simulink model "Trap_Model"  (R2019a)
settings: Solver=FixedStepAuto  StartTime=0.0  StopTime=3  FixedStep=dt  RelTol=1e-3
values from neighbouring files (symbols this model uses):
  disable_droplet_faults = 1    [initTrapModel.m]
  phase_1 = 0    [initMonteCarlo.m]    (also in initTrapModel.m)
  phase_2 = 0.005    [initMonteCarlo.m]    (also in initTrapModel.m)
  Q1 = 0.5*60*1000000000    (= 30000000000)    [initMonteCarlo.m]    (also in initRealModel.m = 2000; initTrapModel.m)
  Q2 = 0.5*60*1000000000    (= 30000000000)    [initMonteCarlo.m]    (also in initRealModel.m = 2000; initTrapModel.m)
  rate_1 = 0.01    [initMonteCarlo.m]    (also in initTrapModel.m)
  rate_2 = 0.01    [initMonteCarlo.m]    (also in initTrapModel.m)
  seed_1 = 0    [initMonteCarlo.m]    (also in initRealModel.m; initTrapModel.m)
  seed_2 = 1    [initMonteCarlo.m]    (also in initRealModel.m; initTrapModel.m)
libraries: simulink x4, SinglePipe_lib x3, Trap_lib x2, Junction_Lib x1
settings Model: Creator=Forest Song  LastModifiedBy=martin

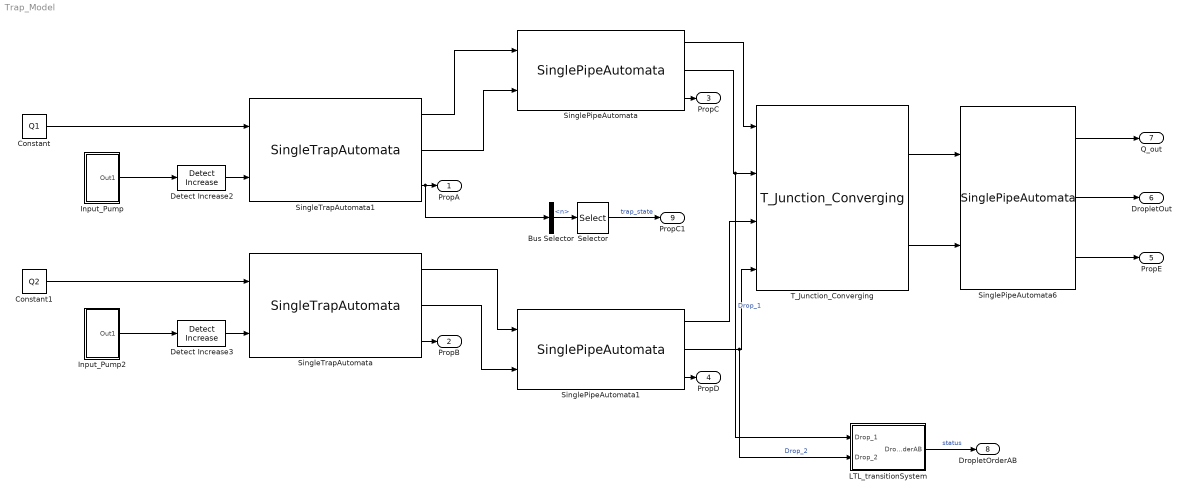
== system Trap_Model ==
  Bus Selector : BusSelector  OutputSignals=n
  Constant : Constant  Value=Q1
  Constant1 : Constant  Value=Q2
  Detect Increase2 : simulink/Logic and Bit Operations/Detect Increase  vinit=0  OutDataTypeStr=boolean
  Detect Increase3 : simulink/Logic and Bit Operations/Detect Increase  vinit=0  OutDataTypeStr=boolean
  Input_Pump : Subsystem  mask{Period=rate_1, Seed=seed_1, PhaseDelay=phase_1}
      mask prompts: Period "droplet rate"; Seed "Simulink:blkprm_prompts:RandNumInitSeed"; PhaseDelay "Simulink:blkprm_prompts:PulseContPhaseDelay"
      mask TypeOptions Period:
      | Pulse
      | Generator/Period
      mask TypeOptions Seed:
      | Uniform Random
      | Number4/Seed
      mask TypeOptions PhaseDelay:
      | Pulse
      | Generator/PhaseDelay
      mask DialogControl Seed Prompt: Seed:
      mask DialogControl PhaseDelay Prompt: Phase delay (secs):
  Input_Pump2 : Subsystem  mask{Period=rate_2, Seed=seed_2, PhaseDelay=phase_2}
      mask prompts: Period "droplet rate"; Seed "Simulink:blkprm_prompts:RandNumInitSeed"; PhaseDelay "Simulink:blkprm_prompts:PulseContPhaseDelay"
      mask TypeOptions Period:
      | Pulse
      | Generator/Period
      mask TypeOptions Seed:
      | Uniform Random
      | Number4/Seed
      mask TypeOptions PhaseDelay:
      | Pulse
      | Generator/PhaseDelay
      mask DialogControl Seed Prompt: Seed:
      mask DialogControl PhaseDelay Prompt: Phase delay (secs):
  LTL_transitionSystem : Subsystem
  Selector : Selector  InputPortWidth=2  IndexOptions=Index vector (dialog)  Indices=[1]  OutputSizes=1
  SinglePipeAutomata : SinglePipe_lib/SinglePipeAutomata  width=W_C  length=L_C  height=H_C  dt=dt
  SinglePipeAutomata1 : SinglePipe_lib/SinglePipeAutomata  width=W_D  length=L_D  height=H_D  dt=dt
  SinglePipeAutomata6 : SinglePipe_lib/SinglePipeAutomata  width=W_E  length=L_E  height=H_E  dt=dt
  SingleTrapAutomata : Trap_lib/SingleTrapAutomata  width=W_B  length=L_B  height=H_B  Rtrap=RTrap  dt=dt
  SingleTrapAutomata1 : Trap_lib/SingleTrapAutomata  width=W_A  length=L_A  height=H_A  Rtrap=RTrap  dt=dt
  T_Junction_Converging : Junction_Lib/T_Junction_Converging  SystemSampleTime=-1
  PropA : Outport
  PropB : Outport  Port=2
  PropC : Outport  Port=3
  PropD : Outport  Port=4
  PropE : Outport  Port=5
  DropletOut : Outport  Port=6
  Q_out : Outport  Port=7
  DropletOrderAB : Outport  Port=8
  PropC1 : Outport  Port=9
  wires:
  Constant1/1 -> SingleTrapAutomata/1
  SingleTrapAutomata1/2 -> SinglePipeAutomata/2
  SingleTrapAutomata/2 -> SinglePipeAutomata1/2
  SingleTrapAutomata/3 -> PropB/1
  SinglePipeAutomata6/1 -> Q_out/1
  SinglePipeAutomata1/3 -> PropD/1
  SinglePipeAutomata1/1 -> T_Junction_Converging/3
  SinglePipeAutomata/1 -> T_Junction_Converging/1
  SinglePipeAutomata/3 -> PropC/1
  T_Junction_Converging/1 -> SinglePipeAutomata6/1
  T_Junction_Converging/2 -> SinglePipeAutomata6/2
  SingleTrapAutomata1/1 -> SinglePipeAutomata/1
  SingleTrapAutomata1/3 -> Bus Selector/1, PropA/1
  SinglePipeAutomata6/2 -> DropletOut/1
  SingleTrapAutomata/1 -> SinglePipeAutomata1/1
  Constant/1 -> SingleTrapAutomata1/1
  Detect Increase2/1 -> SingleTrapAutomata1/2
  Input_Pump/1(Out1) -> Detect Increase2/1
  Input_Pump2/1(Out1) -> Detect Increase3/1
  Detect Increase3/1 -> SingleTrapAutomata/2
  SinglePipeAutomata6/3 -> PropE/1
  LTL_transitionSystem/1(DropletOrderAB) -> DropletOrderAB/1  "status"
  SinglePipeAutomata1/2 -> LTL_transitionSystem/2(Drop_2), T_Junction_Converging/4  "Drop_2"
  SinglePipeAutomata/2 -> LTL_transitionSystem/1(Drop_1), T_Junction_Converging/2  "Drop_1"
  Bus Selector/1 -> Selector/1  "<n>"
  Selector/1 -> PropC1/1  "trap_state"

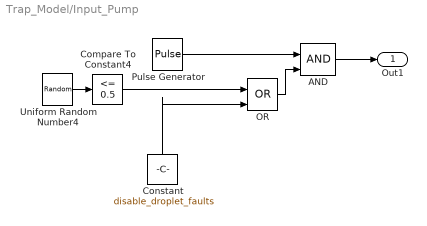
== system Trap_Model/Input_Pump ==
  AND : Logic  IconShape=distinctive  AllPortsSameDT=off  OutDataTypeStr=boolean
  Compare To Constant4 : simulink/Logic and Bit Operations/Compare To Constant  relop=<=  const=0.5  OutDataTypeStr=boolean
  Constant : Constant  Value=disable_droplet_faults
  OR : Logic  Operator=OR  IconShape=distinctive  AllPortsSameDT=off  OutDataTypeStr=boolean
  Pulse Generator : DiscretePulseGenerator  PulseType=Time based  Period=Period  PulseWidth=50  PhaseDelay=PhaseDelay
  Uniform Random Number4 : UniformRandomNumber  Seed=Seed  SampleTime=0.001
  Out1 : Outport
  wires:
  Uniform Random Number4/1 -> Compare To Constant4/1
  Compare To Constant4/1 -> OR/1
  AND/1 -> Out1/1
  Pulse Generator/1 -> AND/1
  OR/1 -> AND/2
  Constant/1 -> OR/2

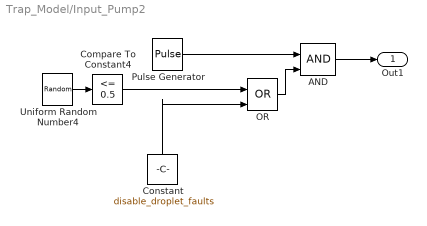
== system Trap_Model/Input_Pump2 ==
  AND : Logic  IconShape=distinctive  AllPortsSameDT=off  OutDataTypeStr=boolean
  Compare To Constant4 : simulink/Logic and Bit Operations/Compare To Constant  relop=<=  const=0.5  OutDataTypeStr=boolean
  Constant : Constant  Value=disable_droplet_faults
  OR : Logic  Operator=OR  IconShape=distinctive  AllPortsSameDT=off  OutDataTypeStr=boolean
  Pulse Generator : DiscretePulseGenerator  PulseType=Time based  Period=Period  PulseWidth=50  PhaseDelay=PhaseDelay
  Uniform Random Number4 : UniformRandomNumber  Seed=Seed  SampleTime=0.001
  Out1 : Outport
  wires:
  OR/1 -> AND/2
  Uniform Random Number4/1 -> Compare To Constant4/1
  Compare To Constant4/1 -> OR/1
  AND/1 -> Out1/1
  Constant/1 -> OR/2
  Pulse Generator/1 -> AND/1

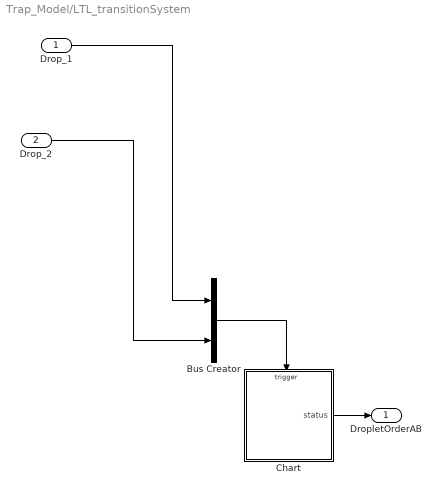
== system Trap_Model/LTL_transitionSystem ==
  Drop_1 : Inport
  Drop_2 : Inport  Port=2
  Bus Creator : BusCreator  Inputs=2
  Chart : Stateflow chart  BlockKeywords=__PRM__SERIALIZED__DATA__:Stateflow Chart,Stateflow Diagram  TreatAsAtomicUnit=on
  DropletOrderAB : Outport
  wires:
  Bus Creator/1 -> Chart/Trigger
  Chart/1(status) -> DropletOrderAB/1
  Drop_2/1 -> Bus Creator/2
  Drop_1/1 -> Bus Creator/1

== stateflow chart Trap_Model/LTL_transitionSystem/Chart ==
  state null
    en:status=0;
  state State_A
    en:status=1;
  state Error
    en:status=2;
  state State_B
    en:status=1;
  (default) -> null [order 3]
  (default) -> State_A [order 1] : Drop_1
  null -> State_A [order 1] : Drop_1
  State_A -> State_B [order 1] : Drop_2
  Error -> State_A [order 1] : Drop_1
  State_A -> Error [order 2] : Drop_1
  State_B -> State_A [order 1] : Drop_1
  null -> State_B [order 2] : Drop_2
  (default) -> State_B [order 2] : Drop_2
  Error -> State_B [order 2] : Drop_2
  State_B -> Error [order 2] : Drop_2
  data: status output =-1
  events: Drop_1 input RISING_EDGE_EVENT; Drop_2 input RISING_EDGE_EVENT
